simulink model "HaloSim_SD"  (R2019b)
settings: Solver=ode45  StartTime=0.0  StopTime=simTime  FixedStep=10^-4  RelTol=1e-4
values from neighbouring files (symbols this model uses):
  A = [zeros(3) eye(3); A21 A22]    [init.m]
  a = zeros(2,1)    [init.m]    (also in new_planner_computation.m)
  b = zeros(2,1)    [init.m]    (also in new_planner_computation.m)
  c = zeros(2,1)    [init.m]    (also in new_planner_computation.m)
  delta = 0.05    [init.m]
  disturbance = 1    [init.m]
  G = [zeros(3); eye(3)]    [init.m]
  K = place(A,G,pole)    [init.m]
  k = 0.1    [init.m]    (also in new_planner_computation.m)
  L2 = 1.1556    [init.m]    (also in new_planner_computation.m)
  mu = 0.012149    [init.m]    (also in new_planner_computation.m)
  Omega = 1.8636    [init.m]    (also in new_planner_computation.m)
  Omega_z = Omega    (= 1.8636)    [init.m]    (also in new_planner_computation.m)
  phi = 0    [init.m]    (also in new_planner_computation.m)
  satValue = inf    [init.m]
  x0 = [L2;0;0;0;0;0]    [init.m]
libraries: sdolib x2
settings Model: Creator=mohd-  LastModifiedBy=mohd-

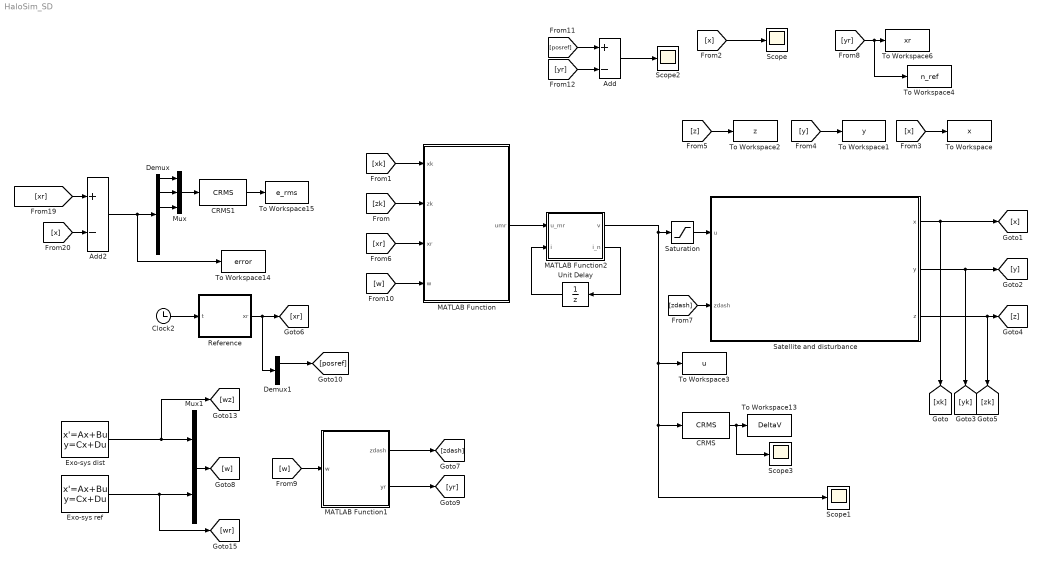
== system HaloSim_SD ==
  Add : Sum  Inputs=+-
  Add2 : Sum  Inputs=+-
  CRMS : sdolib/RMS Blocks/CRMS
      settings: SourceProductName=Simulink Design Optimization  SourceProductBaseCode=SO
  CRMS1 : sdolib/RMS Blocks/CRMS
      settings: SourceProductName=Simulink Design Optimization  SourceProductBaseCode=SO
  Clock2 : Clock
  Demux : Demux  Outputs=6
  Demux1 : Demux  Outputs=[3 3]
  Exo-sys dist : StateSpace  A=[0 -1;1 0]  B=[0;0]  C=eye(2)  D=zeros(2,1)  InitialCondition=[1;0]
  "Exo-sys ref " : StateSpace  A=[0 -Omega;Omega 0]  B=[0;0]  C=eye(2)  D=zeros(2,1)  InitialCondition=[1;0]
  MATLAB Function : MATLAB Function  TreatAsAtomicUnit=on  SystemSampleTime=2*delta
  MATLAB Function1 : MATLAB Function  TreatAsAtomicUnit=on
  MATLAB Function2 : MATLAB Function  TreatAsAtomicUnit=on  SystemSampleTime=delta
  Mux : Mux  Inputs=3
  Mux1 : Mux  Inputs=2
  Reference : MATLAB Function  TreatAsAtomicUnit=on
  Satellite and disturbance : Subsystem
  Saturation : Saturate  UpperLimit=satValue  LowerLimit=-satValue
  Scope{,1..3} (4 alike) : Scope
  To Workspace : ToWorkspace  VariableName=x  SampleTime=10^-3
  To Workspace1 : ToWorkspace  VariableName=y  SampleTime=10^-3
  To Workspace13 : ToWorkspace  VariableName=DeltaV  SampleTime=10^-3
  To Workspace14 : ToWorkspace  VariableName=error  SampleTime=10^-3
  To Workspace15 : ToWorkspace  VariableName=e_rms  SampleTime=delta
  To Workspace2 : ToWorkspace  VariableName=z  SampleTime=10^-3
  To Workspace3 : ToWorkspace  VariableName=u  SampleTime=10^-3
  To Workspace4 : ToWorkspace  VariableName=n_ref  SampleTime=10^-3
  To Workspace6 : ToWorkspace  VariableName=xr  SampleTime=10^-3
  Unit Delay : UnitDelay  InitialCondition=1  SampleTime=delta  HasFrameUpgradeWarning=on
  wires:
  Clock2/1 -> Reference/1(t)
  Satellite and disturbance/1(x) -> [xk], [x]
  Satellite and disturbance/2(y) -> [yk], [y]
  Satellite and disturbance/3(z) -> [zk], [z]
  MATLAB Function/1(umr) -> MATLAB Function2/1(u_mr)
  Unit Delay/1 -> MATLAB Function2/2(i)
  MATLAB Function2/2(i_n) -> Unit Delay/1
  [zk] -> MATLAB Function/2(zk)
  [xk] -> MATLAB Function/1(xk)
  [x] -> Scope/1
  [yr] -> To Workspace4/1, To Workspace6/1
  [y] -> To Workspace1/1
  [z] -> To Workspace2/1
  [x] -> To Workspace/1
  Demux/3 -> Mux/3
  CRMS1/1 -> To Workspace15/1
  Mux/1 -> CRMS1/1
  Demux/2 -> Mux/2
  [xr] -> Add2/1
  Add2/1 -> To Workspace14/1, Demux/1
  [x] -> Add2/2
  Demux/1 -> Mux/1
  MATLAB Function2/1(v) -> Scope1/1, CRMS/1, To Workspace3/1, Saturation/1
  CRMS/1 -> To Workspace13/1, Scope3/1
  Saturation/1 -> Satellite and disturbance/1(u)
  [xr] -> MATLAB Function/3(xr)
  "Exo-sys ref "/1 -> [wr], Mux1/2
  Exo-sys dist/1 -> [wz], Mux1/1
  Mux1/1 -> [w]
  [w] -> MATLAB Function1/1(w)
  MATLAB Function1/2(yr) -> [yr]
  MATLAB Function1/1(zdash) -> [zdash]
  [zdash] -> Satellite and disturbance/2("zdash ")
  [w] -> MATLAB Function/4(w)
  [yr] -> Add/2
  Add/1 -> Scope2/1
  [posref] -> Add/1
  Reference/1(xr) -> Demux1/1, [xr]
  Demux1/1 -> [posref]

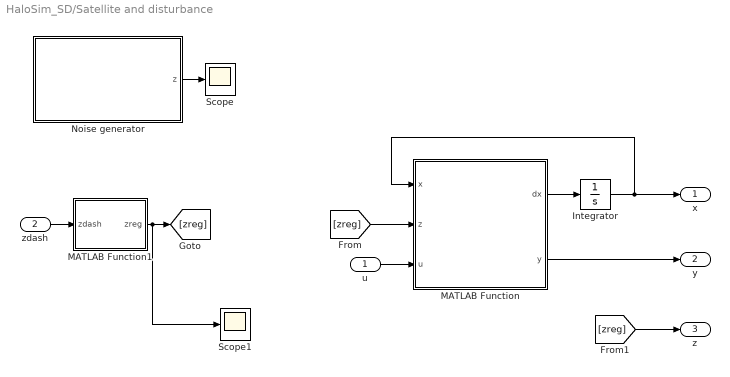
== system HaloSim_SD/Satellite and disturbance ==
  u : Inport
  "zdash " : Inport  Port=2
  Integrator : Integrator  InitialCondition=x0
  MATLAB Function : MATLAB Function  TreatAsAtomicUnit=on
  MATLAB Function1 : MATLAB Function  TreatAsAtomicUnit=on
  Noise generator : Subsystem
  Scope : Scope
  Scope1 : Scope
  x : Outport
  y : Outport  Port=2
  z : Outport  Port=3
  wires:
  Integrator/1 -> x/1, MATLAB Function/1(x)
  MATLAB Function/1(dx) -> Integrator/1
  MATLAB Function/2(y) -> y/1
  u/1 -> MATLAB Function/3(u)
  "zdash "/1 -> MATLAB Function1/1(zdash)
  [zreg] -> MATLAB Function/2(z)
  MATLAB Function1/1(zreg) -> Scope1/1, [zreg]
  [zreg] -> z/1
  Noise generator/1(z) -> Scope/1

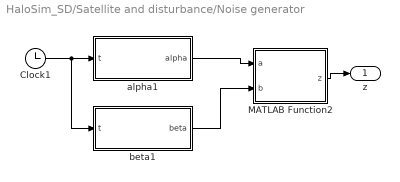
== system HaloSim_SD/Satellite and disturbance/Noise generator ==
  Clock1 : Clock
  MATLAB Function2 : MATLAB Function  TreatAsAtomicUnit=on
  alpha1 : MATLAB Function  TreatAsAtomicUnit=on
  beta1 : MATLAB Function  TreatAsAtomicUnit=on
  z : Outport
  wires:
  Clock1/1 -> beta1/1(t), alpha1/1(t)
  beta1/1(beta) -> MATLAB Function2/2(b)
  alpha1/1(alpha) -> MATLAB Function2/1(a)
  MATLAB Function2/1(z) -> z/1

== matlab function HaloSim_SD/MATLAB Function ==
  data: xk input; umr output; zk input; xr input; mu parameter; delta parameter; w input; A parameter; G parameter; K parameter; L2 parameter; disturbance parameter; Omega parameter; b parameter; a parameter; e parameter; k parameter; c parameter
function umr = mrcontrol(xk,zk,xr, mu,delta, w, A, G, K, L2, disturbance, Omega, b, a, e, k, c)
%umr = [0 0;0 0;0 0];

delta_b = delta;
x1 = xk(1:3);
x2 = xk(4:6);

M = [-1 0 0;
    0 -1 0;
    0 0 0];

N = [0 -1 0;
    1 0 0;
    0 0 0];
% zk  = zeros(4,1);
d1r = [-mu - zk(4)/(1-mu);0;0];
d2r = [1-mu + zk(4)/mu;0;0];

ed1 = x1 - d1r;
absed1 = sqrt(ed1(1)^2+ed1(2)^2+ed1(3)^2);
ed2 = x1 - d2r;
absed2 = sqrt(ed2(1)^2+ed2(2)^2+ed2(3)^2);

f1 = x2;
f2 = -M*x1 - 2*N*x2 - (2*M*x1 + 2*N*x2)*zk(1) ...
           - M*x1*zk(2) - N*x1*zk(3) - ed1*(1 - mu)/absed1^3 ...
           - ed2*mu/absed2^3;

f2dash = -M*(x1+delta_b*f1) - 2*N*(x2+delta_b*f2) - (2*M*(x1+delta_b*f1) + 2*N*(x2+delta_b*f2))*zk(1) ...
           - M*(x1+delta_b*f1)*zk(2) - N*(x1+delta_b*f1)*zk(3) - ed1*(1 - mu)/absed1^3 ...
           - ed2*mu/absed2^3;       

R11 = delta_b^2*eye(3);
R21 = delta_b*eye(3)-2*N*(1+zk(1))*delta_b^2;
R22 = delta_b*eye(3);

R = [R11 zeros(3);R21 R22];

Tz = [b(1)*e 0;0 0;0 -b(1)*e;mu*(1-mu)*a(1)*e 0];
Tr = [k*(1-c(1)+Omega^2)/(2*Omega) 0;0 -k;-k 0];
S2 = [0 -Omega;Omega 0];
Seq = [L2;0;0];
if disturbance == 1
    wz = w(1:2);
else
    wz = zeros(2,1);
end
wr = w(3:4);
pi = [-Tr*wr + Seq;-Tr*S2*wr];

F = xk+delta_b*[x2+f1;f2+f2dash]+ [delta_b^2*f2;zeros(3,1)];
%ref = (A-G*K)*xk + G*K*pi;
% PD = exp((A-G*K)*delta_b);
% BD = (PD-eye(size(PD)))*pinv(A-G*K)*G;
% ref = PD*xk + BD*K*pi;
u = pinv(R)*(pi-F);
% u = pinv(R)*(xr-F);
u1 = u(1:3);
u2 = u(4:6);
umr = [u1 u2];

== matlab function HaloSim_SD/Satellite and disturbance/MATLAB Function ==
  data: x input; z input; dx output; u input; y output; mu parameter
function [dx, y] = Satellite(x,z, u, mu)

x1 = x(1:3);
x2 = x(4:6);

M = [-1 0 0;
    0 -1 0;
    0 0 0];

N = [0 -1 0;
    1 0 0;
    0 0 0];

d1r = [-mu - z(4)/(1-mu);0;0];
d2r = [1-mu + z(4)/mu;0;0];

ed1 = x1 - d1r;
absed1 = sqrt(ed1(1)^2+ed1(2)^2+ed1(3)^2);
ed2 = x1 - d2r;
absed2 = sqrt(ed2(1)^2+ed2(2)^2+ed2(3)^2);

f1 = x2;
f2 = -M*x1 - 2*N*x2 - (2*M*x1 + 2*N*x2)*z(1) ...
           - M*x1*z(2) - N*x1*z(3) - ed1*(1 - mu)/absed1^3 ...
           - ed2*mu/absed2^3;
F = [f1; f2];
G = [zeros(3); eye(3)];


dx = F + G*u;
y  = x1;

== matlab function HaloSim_SD/MATLAB Function2 ==
  data: u_mr input; v output; i input size=1; i_n output size=1
function [v,i_n] = fcn(u_mr, i)
if i <2
    i_n = i+1; 
else
    i_n = 1;
end

v = u_mr(:, i);

== matlab function HaloSim_SD/Satellite and disturbance/MATLAB Function1 ==
  data: zdash input; zreg output; disturbance parameter
function zreg = fcn(zdash, disturbance)

if disturbance == 1 
    zreg = zdash;
else
    zreg = zeros(4,1);
end

== matlab function HaloSim_SD/Reference ==
  data: t input; xr output; c parameter; Omega parameter; Omega_z parameter; L2 parameter; k parameter; e parameter
function xr = refer(t,c,Omega,Omega_z,L2,k,e)
%#codegen


Seq = [L2;0;0;0;0;0];
ho1 = [(-k*(1-c(1)+Omega^2)/(2*Omega))*cos(Omega*t);
       k*sin(Omega*t);
       k*cos(Omega_z*t)];
   
diffho1 = [(k*(1-c(1)+Omega^2)/2)*sin(Omega*t);
           Omega*k*cos(Omega*t);
           -Omega_z*k*sin(Omega_z*t)];
      
% Halo orbit reference type 1       
xr = Seq;
xr = xr + [ho1;diffho1];

== matlab function HaloSim_SD/Satellite and disturbance/Noise generator/alpha1 ==
  data: t input; alpha output; a parameter; phi parameter; e parameter
function alpha = a(t,a,phi,e)
%#codegen
a1 = a(1)*e*cos(t+phi);

alpha = a1 + a(2)*e^2*(1+cos(2*(t+phi)));

== matlab function HaloSim_SD/Satellite and disturbance/Noise generator/beta1 ==
  data: t input; beta output; b parameter; phi parameter; e parameter
function beta = b(t,b,phi,e)
%#codegen
b1 = b(1)*e*cos(t+phi);
bd = -b(1)*e*sin(t+phi);

beta = [b1 + b(2)*e^2*(1+cos(2*(t+phi)));
         (1+cos(2*(t+phi)))*e^2*b(1)^2/2;
         bd - 2*b(2)*e^2*sin(2*(t+phi))];

== matlab function HaloSim_SD/Satellite and disturbance/Noise generator/MATLAB Function2 ==
  data: a input; z output; b input; mu parameter; disturbance parameter
function z = z(a,b,mu,disturbance)
%#codegen

if disturbance == 1
    z = [b;mu*(1-mu)*a];
else
    z = zeros(4,1);
end

== matlab function HaloSim_SD/MATLAB Function1 ==
  data: zdash output; w input; yr output; c parameter; Omega parameter; k parameter; a parameter; b parameter; mu parameter; e parameter; L2 parameter
function [zdash,yr] = fcn(w, c, Omega, k, a, b, mu, e, L2)

Seq = [L2;0;0];

T1 = [b(1)*e 0;0 0;0 -b(1)*e;mu*(1-mu)*a(1)*e 0];
Q1 = [k*(1-c(1)+Omega^2)/(2*Omega) 0;0 -k;-k 0];

zdash = T1*w(1:2);
yr = Q1*w(3:4) + Seq;
